simulink model "ParkingMeterSystemNew"  (R2023a)
settings: Solver=FixedStepDiscrete  StartTime=0.0  StopTime=Inf  RelTol=1e-3
PreLoadFcn:
  | % Open the external C# interface
  | startGUI();
PostLoadFcn:
  | warning('off','Simulink:SimulationPacing:UnsupportedSimulationMode');
InitFcn:
  | % Update the sampling time based on the selected simulation mode
  | updateSamplingTime('ParkingMeterSystemNew','SAMPLING_TIME');
undefined symbols (not defined in the file): D1, P
CloseFcn:
  | % Close the external C# interface
  | closeGUI();
settings Model: DataDictionary=Parameters.sldd  Creator=sebas  LastModifiedBy=sebas
settings OptimizationCC: DefaultParameterBehavior=Inlined  EnhancedBackFolding=on  PassReuseOutputArgsAs=Individual arguments  ZeroExternalMemoryAtStartup=off  ZeroInternalMemoryAtStartup=off  OptimizeBlockOrder=speed  DifferentSizesBufferReuse=on  OptimizationCustomize=off  EfficientTunableParamExpr=on
settings DebuggingCC: ParameterTunabilityLossMsg=error
settings SFSimCC: MATLABDynamicMemAlloc=off
settings RTWCC: Description=Embedded Coder  SystemTargetFile=ert.tlc  TemplateMakefile=ert_default_tmf
settings CodeAppCC: ForceParamTrailComments=on  IgnoreCustomStorageClasses=off  MaxIdLength=61  OperatorAnnotations=on  SimulinkDataObjDesc=on  SFDataObjDesc=on  InsertBlockDesc=on
settings ERTTargetCC: TargetLangStandard=C99 (ISO)  GenerateSampleERTMain=on  InlinedParameterPlacement=NonHierarchical  ERTCustomFileTemplate=example_file_process.tlc

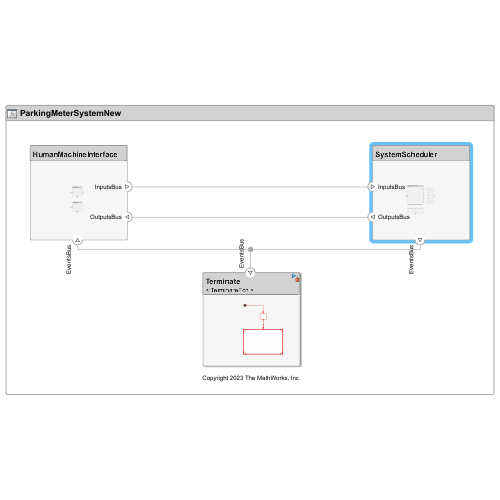
[thumbnail: Simulink's stored preview of the top-level diagram]
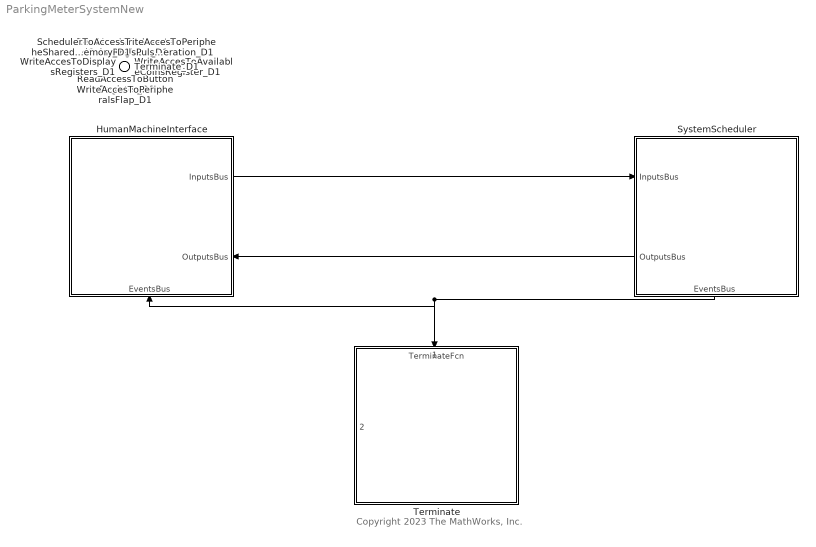
== system ParkingMeterSystemNew ==
  note: Copyright 2023 The MathWorks, Inc.
  ReadAccessToButtonsRegister_D1 : Inport  OutputFunctionCall=on
  ReadAccessToInsertedCoinsRegister_D1 : Inport  Port=2  OutputFunctionCall=on
  WriteAccesToAvailableCoinsRegister_D1 : Inport  Port=3  OutputFunctionCall=on
  WriteAccesToDisplaysRegisters_D1 : Inport  Port=4  OutputFunctionCall=on
  WriteAccesToPeripheralsFlap_D1 : Inport  Port=5  OutputFunctionCall=on
  WriteAccesToPeripheralsPulseGeneration_D1 : Inport  Port=6  OutputFunctionCall=on
  SchedulerToAccessTheSharedMemory_D1 : Inport  Port=7  OutputFunctionCall=on
  Terminate_D1 : Inport  Port=8  OutputFunctionCall=on
  HumanMachineInterface : Subsystem
      settings: PortSchema="{\"entries\":[{\"content\":{\"headerSize\":26,\"margin\":15,\"minimumSpacing\":25,\"sides\":[{\"content\":{},\"type\":\"ConnectorPlacement.EquallySpacedRectSide\",\"uuid\":\"be809503-f1ea-4380-8942-33d79f2ad371\"},{\"content\":{\"connectorIds\":[\"Out1\",\"In2\"],\"side\":\"RIGHT\"},\"type\":\"ConnectorPlacement.EquallySpacedRectSide\",\"uuid\":\"d20c5475-d043-4994-ac49-3eb74728e760\"},{\"content\":{\"side\":\"TOP\"},\"type\":\"ConnectorPlacement.EquallySpacedRectSide\",\"uuid\":\"367a4a40-2fef-41b1-a218-3cfa4d79ed8f\"},{\"content\":{\"connectorIds\":[\"In1\"],\"side\":\"BOTTOM\"},\"type\":\"ConnectorPlacement.EquallySpacedRectSide\",\"uuid\":\"ad45a532-4028-4d32-9ed1-5493ed102a58\"}]},\"type\":\"ConnectorPlacement.EquallySpacedConnector\",\"uuid\":\"eb419f36-354b-4c4e-9a9c-8f8f96d7f82d\"}],\"packageUris\":[\"http://schema.mathworks.com/mf0/Connector/R2020b\"],\"version\":\"1.0\"}"
  SystemScheduler : Subsystem
      settings: PortSchema="{\"entries\":[{\"content\":{\"headerSize\":26,\"margin\":15,\"minimumSpacing\":25,\"sides\":[{\"content\":{\"connectorIds\":[\"In1\",\"Out2\"]},\"type\":\"ConnectorPlacement.EquallySpacedRectSide\",\"uuid\":\"be809503-f1ea-4380-8942-33d79f2ad371\"},{\"content\":{\"side\":\"RIGHT\"},\"type\":\"ConnectorPlacement.EquallySpacedRectSide\",\"uuid\":\"d20c5475-d043-4994-ac49-3eb74728e760\"},{\"content\":{\"side\":\"TOP\"},\"type\":\"ConnectorPlacement.EquallySpacedRectSide\",\"uuid\":\"367a4a40-2fef-41b1-a218-3cfa4d79ed8f\"},{\"content\":{\"connectorIds\":[\"Out1\"],\"side\":\"BOTTOM\"},\"type\":\"ConnectorPlacement.EquallySpacedRectSide\",\"uuid\":\"599a3aa0-021a-4e17-bee6-5fef34730978\"}]},\"type\":\"ConnectorPlacement.EquallySpacedConnector\",\"uuid\":\"eb419f36-354b-4c4e-9a9c-8f8f96d7f82d\"}],\"packageUris\":[\"http://schema.mathworks.com/mf0/Connector/R2020b\"],\"version\":\"1.0\"}"
  Terminate : ModelReference  ModelNameDialog=TerminateFcn  SimulationMode=Normal  ScheduleRates=on  CachedPortDiscreteRates=[0.001]  ModelEventPortInfo=P:D1[0.001][0][0]  ModelReferenceVersion=8.4
      settings: PortSchema="{\"entries\":[{\"content\":{\"headerSize\":38,\"margin\":15,\"minimumSpacing\":25,\"sides\":[{\"content\":{},\"type\":\"ConnectorPlacement.EquallySpacedRectSide\",\"uuid\":\"be809503-f1ea-4380-8942-33d79f2ad371\"},{\"content\":{\"side\":\"RIGHT\"},\"type\":\"ConnectorPlacement.EquallySpacedRectSide\",\"uuid\":\"d20c5475-d043-4994-ac49-3eb74728e760\"},{\"content\":{\"connectorIds\":[\"In1\"],\"side\":\"TOP\"},\"type\":\"ConnectorPlacement.EquallySpacedRectSide\",\"uuid\":\"367a4a40-2fef-41b1-a218-3cfa4d79ed8f\"},{\"content\":{\"connectorIds\":[\"In2\"],\"side\":\"HIDDEN\"},\"type\":\"ConnectorPlacement.EquallySpacedRectSide\",\"uuid\":\"2b7aa608-e8c7-4427-8225-0280e4f358e9\"}]},\"type\":\"ConnectorPlacement.EquallySpacedConnector\",\"uuid\":\"eb419f36-354b-4c4e-9a9c-8f8f96d7f82d\"}],\"packageUris\":[\"http://schema.mathworks.com/mf0/Connector/R2020b\"],\"version\":\"1.0\"}"
  wires:
  SystemScheduler/2(OutputsBus) -> HumanMachineInterface/2(OutputsBus)
  HumanMachineInterface/1(InputsBus) -> SystemScheduler/1(InputsBus)
  SystemScheduler/1(EventsBus) -> Terminate/1, HumanMachineInterface/1(EventsBus)

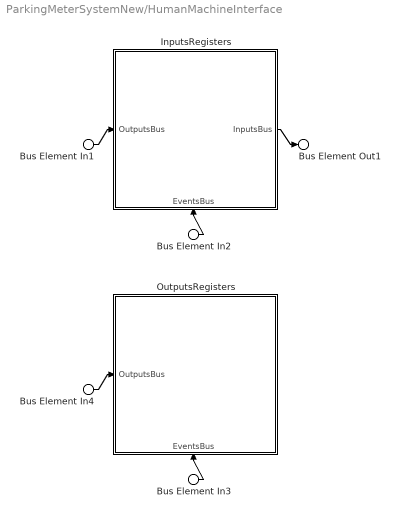
== system ParkingMeterSystemNew/HumanMachineInterface ==
  Bus Element In2 : Inport  PortName=EventsBus
  Bus Element In3 : Inport  PortName=EventsBus
  Bus Element In1 : Inport  Port=2  PortName=OutputsBus
  Bus Element In4 : Inport  Port=2  PortName=OutputsBus
  InputsRegisters : Subsystem
      settings: PortSchema="{\"entries\":[{\"content\":{\"headerSize\":26,\"margin\":15,\"minimumSpacing\":25,\"sides\":[{\"content\":{\"connectorIds\":[\"In2\"]},\"type\":\"ConnectorPlacement.EquallySpacedRectSide\",\"uuid\":\"be809503-f1ea-4380-8942-33d79f2ad371\"},{\"content\":{\"connectorIds\":[\"Out1\"],\"side\":\"RIGHT\"},\"type\":\"ConnectorPlacement.EquallySpacedRectSide\",\"uuid\":\"d20c5475-d043-4994-ac49-3eb74728e760\"},{\"content\":{\"side\":\"TOP\"},\"type\":\"ConnectorPlacement.EquallySpacedRectSide\",\"uuid\":\"367a4a40-2fef-41b1-a218-3cfa4d79ed8f\"},{\"content\":{\"connectorIds\":[\"In1\"],\"side\":\"BOTTOM\"},\"type\":\"ConnectorPlacement.EquallySpacedRectSide\",\"uuid\":\"42433694-7d38-411e-8c36-0d107f91df78\"}]},\"type\":\"ConnectorPlacement.EquallySpacedConnector\",\"uuid\":\"eb419f36-354b-4c4e-9a9c-8f8f96d7f82d\"}],\"packageUris\":[\"http://schema.mathworks.com/mf0/Connector/R2020b\"],\"version\":\"1.0\"}"
  OutputsRegisters : Subsystem
      settings: PortSchema="{\"entries\":[{\"content\":{\"headerSize\":26,\"margin\":15,\"minimumSpacing\":25,\"sides\":[{\"content\":{\"connectorIds\":[\"In1\"]},\"type\":\"ConnectorPlacement.EquallySpacedRectSide\",\"uuid\":\"be809503-f1ea-4380-8942-33d79f2ad371\"},{\"content\":{\"side\":\"RIGHT\"},\"type\":\"ConnectorPlacement.EquallySpacedRectSide\",\"uuid\":\"d20c5475-d043-4994-ac49-3eb74728e760\"},{\"content\":{\"side\":\"TOP\"},\"type\":\"ConnectorPlacement.EquallySpacedRectSide\",\"uuid\":\"367a4a40-2fef-41b1-a218-3cfa4d79ed8f\"},{\"content\":{\"connectorIds\":[\"In2\"],\"side\":\"BOTTOM\"},\"type\":\"ConnectorPlacement.EquallySpacedRectSide\",\"uuid\":\"9411f4e0-b09e-492c-9d7b-7970a952076c\"}]},\"type\":\"ConnectorPlacement.EquallySpacedConnector\",\"uuid\":\"eb419f36-354b-4c4e-9a9c-8f8f96d7f82d\"}],\"packageUris\":[\"http://schema.mathworks.com/mf0/Connector/R2020b\"],\"version\":\"1.0\"}"
  Bus Element Out1 : Outport  PortName=InputsBus
  wires:
  Bus Element In1/1 -> InputsRegisters/2(OutputsBus)
  InputsRegisters/1(InputsBus) -> Bus Element Out1/1
  Bus Element In2/1 -> InputsRegisters/1(EventsBus)
  Bus Element In3/1 -> OutputsRegisters/2(EventsBus)
  Bus Element In4/1 -> OutputsRegisters/1(OutputsBus)

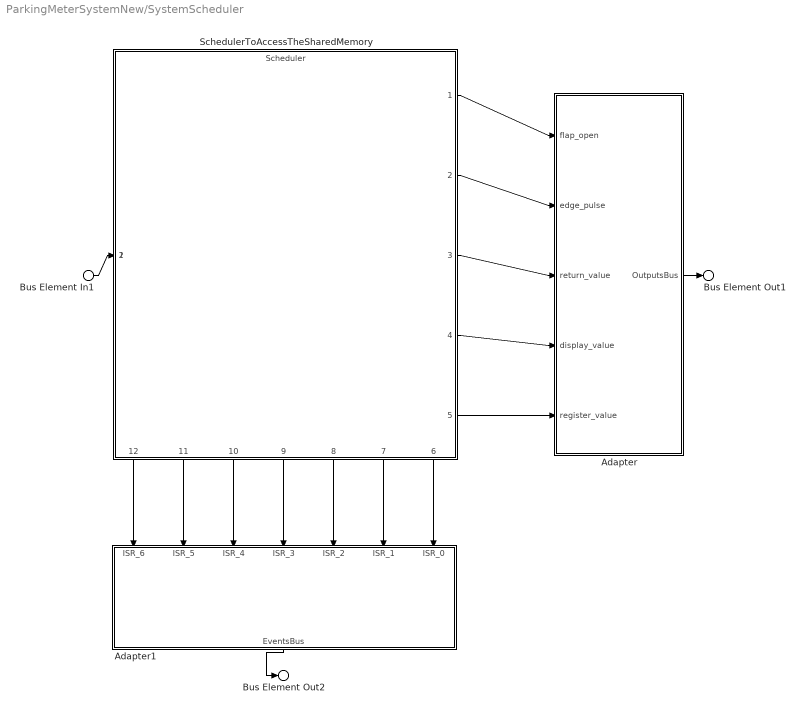
== system ParkingMeterSystemNew/SystemScheduler ==
  Bus Element In1 : Inport  PortName=InputsBus
  Adapter : Subsystem
      settings: PortSchema="{\"entries\":[{\"content\":{\"margin\":10,\"minimumSpacing\":15,\"sides\":[{\"content\":{\"connectorIds\":[\"In1\",\"In2\",\"In3\",\"In4\",\"In5\"]},\"type\":\"ConnectorPlacement.EquallySpacedRectSide\",\"uuid\":\"be809503-f1ea-4380-8942-33d79f2ad371\"},{\"content\":{\"connectorIds\":[\"Out1\"],\"side\":\"RIGHT\"},\"type\":\"ConnectorPlacement.EquallySpacedRectSide\",\"uuid\":\"d20c5475-d043-4994-ac49-3eb74728e760\"},{\"content\":{\"side\":\"TOP\"},\"type\":\"ConnectorPlacement.EquallySpacedRectSide\",\"uuid\":\"367a4a40-2fef-41b1-a218-3cfa4d79ed8f\"}]},\"type\":\"ConnectorPlacement.EquallySpacedConnector\",\"uuid\":\"eb419f36-354b-4c4e-9a9c-8f8f96d7f82d\"}],\"packageUris\":[\"http://schema.mathworks.com/mf0/Connector/R2020b\"],\"version\":\"1.0\"}"
  Adapter1 : Subsystem
      settings: PortSchema="{\"entries\":[{\"content\":{\"margin\":10,\"minimumSpacing\":15,\"sides\":[{\"content\":{},\"type\":\"ConnectorPlacement.EquallySpacedRectSide\",\"uuid\":\"be809503-f1ea-4380-8942-33d79f2ad371\"},{\"content\":{\"side\":\"RIGHT\"},\"type\":\"ConnectorPlacement.EquallySpacedRectSide\",\"uuid\":\"d20c5475-d043-4994-ac49-3eb74728e760\"},{\"content\":{\"connectorIds\":[\"In1\",\"In2\",\"In3\",\"In4\",\"In5\",\"In6\",\"In7\"],\"side\":\"TOP\"},\"type\":\"ConnectorPlacement.EquallySpacedRectSide\",\"uuid\":\"367a4a40-2fef-41b1-a218-3cfa4d79ed8f\"},{\"content\":{\"connectorIds\":[\"Out1\"],\"side\":\"BOTTOM\"},\"type\":\"ConnectorPlacement.EquallySpacedRectSide\",\"uuid\":\"de1afc0c-f7fe-45f0-a616-bbe694a265ab\"}]},\"type\":\"ConnectorPlacement.EquallySpacedConnector\",\"uuid\":\"eb419f36-354b-4c4e-9a9c-8f8f96d7f82d\"}],\"packageUris\":[\"http://schema.mathworks.com/mf0/Connector/R2020b\"],\"version\":\"1.0\"}"
  SchedulerToAccessTheSharedMemory : ModelReference  ModelNameDialog=Scheduler  SimulationMode=Normal  ScheduleRates=on  CachedPortDiscreteRates=[0.001]  ModelEventPortInfo=P:D1[0.001][0][0]  ModelReferenceVersion=8.3
      settings: PortSchema="{\"entries\":[{\"content\":{\"headerSize\":38,\"margin\":15,\"minimumSpacing\":25,\"sides\":[{\"content\":{\"connectorIds\":[\"In1\"]},\"type\":\"ConnectorPlacement.EquallySpacedRectSide\",\"uuid\":\"be809503-f1ea-4380-8942-33d79f2ad371\"},{\"content\":{\"connectorIds\":[\"Out1\",\"Out2\",\"Out3\",\"Out4\",\"Out5\"],\"side\":\"RIGHT\"},\"type\":\"ConnectorPlacement.EquallySpacedRectSide\",\"uuid\":\"d20c5475-d043-4994-ac49-3eb74728e760\"},{\"content\":{\"side\":\"TOP\"},\"type\":\"ConnectorPlacement.EquallySpacedRectSide\",\"uuid\":\"367a4a40-2fef-41b1-a218-3cfa4d79ed8f\"},{\"content\":{\"connectorIds\":[\"Out12\",\"Out11\",\"Out10\",\"Out9\",\"Out8\",\"Out7\",\"Out6\"],\"side\":\"BOTTOM\"},\"type\":\"ConnectorPlacement.EquallySpacedRectSide\",\"uuid\":\"fb86e00b-f9c7-4f3f-8cbd-dd4de8ac92df\"},{\"content\":{\"connectorIds\":[\"In2\"],\"side\":\"HIDDEN\"},\"type\":\"ConnectorPlacement.EquallySpacedRectSide\",\"uuid\":\"74e265bb-5a4f-4039-8bd9-f78af680f503\"}]},\"type\":\"ConnectorPlacement.EquallySpacedConnector\",\"uuid\":\"eb419f36-354b-4c4e-9a9c-8f8f96d7f82d\"}],\"packageUris\":[\"http://schema.mathworks.com/mf0/Connector/R2020b\"],\"version\":\"1.0\"}"
  Bus Element Out2 : Outport  PortName=EventsBus
  Bus Element Out1 : Outport  Port=2  PortName=OutputsBus
  wires:
  Adapter/1(OutputsBus) -> Bus Element Out1/1
  SchedulerToAccessTheSharedMemory/1 -> Adapter/1(flap_open)
  SchedulerToAccessTheSharedMemory/2 -> Adapter/2(edge_pulse)
  SchedulerToAccessTheSharedMemory/3 -> Adapter/3(return_value)
  SchedulerToAccessTheSharedMemory/4 -> Adapter/4(display_value)
  SchedulerToAccessTheSharedMemory/5 -> Adapter/5(register_value)
  Adapter1/1(EventsBus) -> Bus Element Out2/1
  SchedulerToAccessTheSharedMemory/12 -> Adapter1/1(ISR_6)
  SchedulerToAccessTheSharedMemory/11 -> Adapter1/2(ISR_5)
  SchedulerToAccessTheSharedMemory/10 -> Adapter1/3(ISR_4)
  SchedulerToAccessTheSharedMemory/9 -> Adapter1/4(ISR_3)
  SchedulerToAccessTheSharedMemory/8 -> Adapter1/5(ISR_2)
  SchedulerToAccessTheSharedMemory/7 -> Adapter1/6(ISR_1)
  SchedulerToAccessTheSharedMemory/6 -> Adapter1/7(ISR_0)
  Bus Element In1/1 -> SchedulerToAccessTheSharedMemory/1

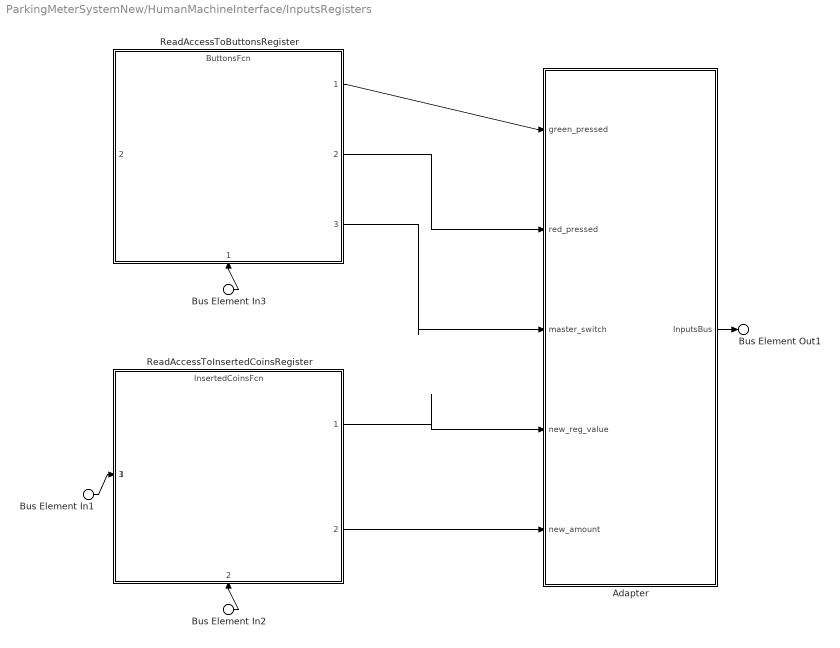
== system ParkingMeterSystemNew/HumanMachineInterface/InputsRegisters ==
  Bus Element In2 : Inport  PortName=EventsBus
  Bus Element In3 : Inport  PortName=EventsBus
  Bus Element In1 : Inport  Port=2  PortName=OutputsBus
  Adapter : Subsystem
      settings: PortSchema="{\"entries\":[{\"content\":{\"margin\":10,\"minimumSpacing\":15,\"sides\":[{\"content\":{\"connectorIds\":[\"In1\",\"In2\",\"In3\",\"In4\",\"In5\"]},\"type\":\"ConnectorPlacement.EquallySpacedRectSide\",\"uuid\":\"be809503-f1ea-4380-8942-33d79f2ad371\"},{\"content\":{\"connectorIds\":[\"Out1\"],\"side\":\"RIGHT\"},\"type\":\"ConnectorPlacement.EquallySpacedRectSide\",\"uuid\":\"d20c5475-d043-4994-ac49-3eb74728e760\"},{\"content\":{\"side\":\"TOP\"},\"type\":\"ConnectorPlacement.EquallySpacedRectSide\",\"uuid\":\"367a4a40-2fef-41b1-a218-3cfa4d79ed8f\"}]},\"type\":\"ConnectorPlacement.EquallySpacedConnector\",\"uuid\":\"eb419f36-354b-4c4e-9a9c-8f8f96d7f82d\"}],\"packageUris\":[\"http://schema.mathworks.com/mf0/Connector/R2020b\"],\"version\":\"1.0\"}"
  ReadAccessToButtonsRegister : ModelReference  ModelNameDialog=ButtonsFcn  SimulationMode=Normal  ScheduleRates=on  CachedPortDiscreteRates=[0.001]  ModelEventPortInfo=P:D1[0.001][0][0]  ModelReferenceVersion=8.1
      settings: PortSchema="{\"entries\":[{\"content\":{\"headerSize\":38,\"margin\":15,\"minimumSpacing\":25,\"sides\":[{\"content\":{},\"type\":\"ConnectorPlacement.EquallySpacedRectSide\",\"uuid\":\"be809503-f1ea-4380-8942-33d79f2ad371\"},{\"content\":{\"connectorIds\":[\"Out1\",\"Out2\",\"Out3\"],\"side\":\"RIGHT\"},\"type\":\"ConnectorPlacement.EquallySpacedRectSide\",\"uuid\":\"d20c5475-d043-4994-ac49-3eb74728e760\"},{\"content\":{\"side\":\"TOP\"},\"type\":\"ConnectorPlacement.EquallySpacedRectSide\",\"uuid\":\"367a4a40-2fef-41b1-a218-3cfa4d79ed8f\"},{\"content\":{\"connectorIds\":[\"In1\"],\"side\":\"BOTTOM\"},\"type\":\"ConnectorPlacement.EquallySpacedRectSide\",\"uuid\":\"20a3fabb-dc20-4c8a-b758-ffeffe12cb5d\"},{\"content\":{\"connectorIds\":[\"In2\"],\"side\":\"HIDDEN\"},\"type\":\"ConnectorPlacement.EquallySpacedRectSide\",\"uuid\":\"619db0d7-0664-4085-915a-a74ff553ccfa\"}]},\"type\":\"ConnectorPlacement.EquallySpacedConnector\",\"uuid\":\"eb419f36-354b-4c4e-9a9c-8f8f96d7f82d\"}],\"packageUris\":[\"http://schema.mathworks.com/mf0/Connector/R2020b\"],\"version\":\"1.0\"}"
  ReadAccessToInsertedCoinsRegister : ModelReference  ModelNameDialog=InsertedCoinsFcn  SimulationMode=Normal  ScheduleRates=on  CachedPortDiscreteRates=[0.001]  ModelEventPortInfo=P:D1[0.001][0][0]  ModelReferenceVersion=8.4
      settings: PortSchema="{\"entries\":[{\"content\":{\"headerSize\":38,\"margin\":15,\"minimumSpacing\":25,\"sides\":[{\"content\":{\"connectorIds\":[\"In1\"]},\"type\":\"ConnectorPlacement.EquallySpacedRectSide\",\"uuid\":\"be809503-f1ea-4380-8942-33d79f2ad371\"},{\"content\":{\"connectorIds\":[\"Out1\",\"Out2\"],\"side\":\"RIGHT\"},\"type\":\"ConnectorPlacement.EquallySpacedRectSide\",\"uuid\":\"d20c5475-d043-4994-ac49-3eb74728e760\"},{\"content\":{\"side\":\"TOP\"},\"type\":\"ConnectorPlacement.EquallySpacedRectSide\",\"uuid\":\"367a4a40-2fef-41b1-a218-3cfa4d79ed8f\"},{\"content\":{\"connectorIds\":[\"In2\"],\"side\":\"BOTTOM\"},\"type\":\"ConnectorPlacement.EquallySpacedRectSide\",\"uuid\":\"c4a18945-d859-4bf0-a176-342256d1a336\"},{\"content\":{\"connectorIds\":[\"In3\"],\"side\":\"HIDDEN\"},\"type\":\"ConnectorPlacement.EquallySpacedRectSide\",\"uuid\":\"52804af8-db2a-4760-b62b-c289e870e5aa\"}]},\"type\":\"ConnectorPlacement.EquallySpacedConnector\",\"uuid\":\"eb419f36-354b-4c4e-9a9c-8f8f96d7f82d\"}],\"packageUris\":[\"http://schema.mathworks.com/mf0/Connector/R2020b\"],\"version\":\"1.0\"}"
  Bus Element Out1 : Outport  PortName=InputsBus
  wires:
  Bus Element In1/1 -> ReadAccessToInsertedCoinsRegister/1
  Bus Element In2/1 -> ReadAccessToInsertedCoinsRegister/2
  Bus Element In3/1 -> ReadAccessToButtonsRegister/1
  Adapter/1(InputsBus) -> Bus Element Out1/1
  ReadAccessToButtonsRegister/1 -> Adapter/1(green_pressed)
  ReadAccessToButtonsRegister/2 -> Adapter/2(red_pressed)
  ReadAccessToButtonsRegister/3 -> Adapter/3(master_switch)
  ReadAccessToInsertedCoinsRegister/1 -> Adapter/4(new_reg_value)
  ReadAccessToInsertedCoinsRegister/2 -> Adapter/5(new_amount)

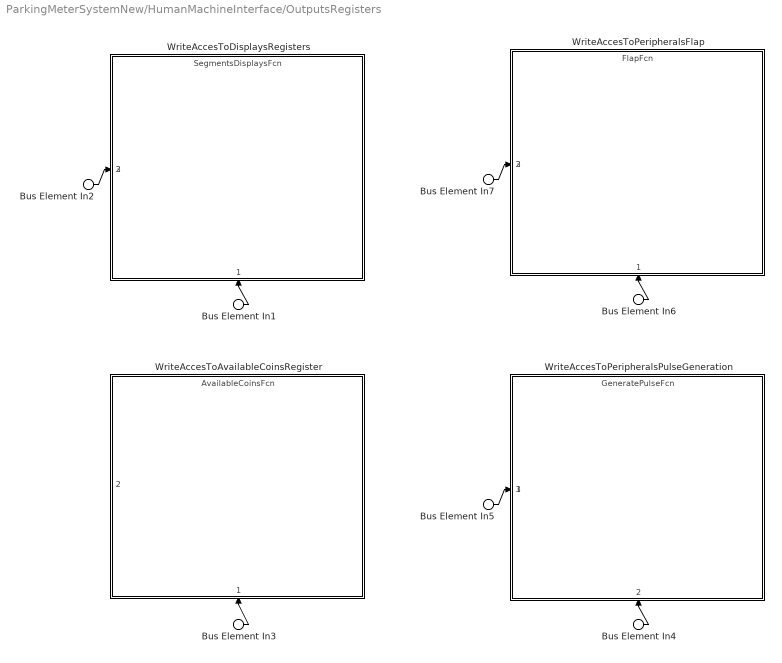
== system ParkingMeterSystemNew/HumanMachineInterface/OutputsRegisters ==
  Bus Element In2 : Inport  PortName=OutputsBus
  Bus Element In5 : Inport  PortName=OutputsBus
  Bus Element In7 : Inport  PortName=OutputsBus
  Bus Element In{1,3..4,6} (4 alike) : Inport  Port=2  PortName=EventsBus
  WriteAccesToAvailableCoinsRegister : ModelReference  ModelNameDialog=AvailableCoinsFcn  SimulationMode=Normal  ScheduleRates=on  CachedPortDiscreteRates=[0.001]  ModelEventPortInfo=P:D1[0.001][0][0]  ModelReferenceVersion=8.4
      settings: PortSchema="{\"entries\":[{\"content\":{\"headerSize\":38,\"margin\":15,\"minimumSpacing\":25,\"sides\":[{\"content\":{},\"type\":\"ConnectorPlacement.EquallySpacedRectSide\",\"uuid\":\"be809503-f1ea-4380-8942-33d79f2ad371\"},{\"content\":{\"side\":\"RIGHT\"},\"type\":\"ConnectorPlacement.EquallySpacedRectSide\",\"uuid\":\"d20c5475-d043-4994-ac49-3eb74728e760\"},{\"content\":{\"side\":\"TOP\"},\"type\":\"ConnectorPlacement.EquallySpacedRectSide\",\"uuid\":\"367a4a40-2fef-41b1-a218-3cfa4d79ed8f\"},{\"content\":{\"connectorIds\":[\"In1\"],\"side\":\"BOTTOM\"},\"type\":\"ConnectorPlacement.EquallySpacedRectSide\",\"uuid\":\"0ec21bd5-d732-4e1f-9584-045b5c892f8a\"},{\"content\":{\"connectorIds\":[\"In2\"],\"side\":\"HIDDEN\"},\"type\":\"ConnectorPlacement.EquallySpacedRectSide\",\"uuid\":\"3eb33428-824a-4da5-832a-2eacaca34f61\"}]},\"type\":\"ConnectorPlacement.EquallySpacedConnector\",\"uuid\":\"eb419f36-354b-4c4e-9a9c-8f8f96d7f82d\"}],\"packageUris\":[\"http://schema.mathworks.com/mf0/Connector/R2020b\"],\"version\":\"1.0\"}"
  WriteAccesToDisplaysRegisters : ModelReference  ModelNameDialog=SegmentsDisplaysFcn  SimulationMode=Normal  ScheduleRates=on  CachedPortDiscreteRates=[0.001]  ModelEventPortInfo=P:D1[0.001][0][0]  ModelReferenceVersion=8.4
      settings: PortSchema="{\"entries\":[{\"content\":{\"headerSize\":38,\"margin\":15,\"minimumSpacing\":25,\"sides\":[{\"content\":{\"connectorIds\":[\"In2\"]},\"type\":\"ConnectorPlacement.EquallySpacedRectSide\",\"uuid\":\"be809503-f1ea-4380-8942-33d79f2ad371\"},{\"content\":{\"side\":\"RIGHT\"},\"type\":\"ConnectorPlacement.EquallySpacedRectSide\",\"uuid\":\"d20c5475-d043-4994-ac49-3eb74728e760\"},{\"content\":{\"side\":\"TOP\"},\"type\":\"ConnectorPlacement.EquallySpacedRectSide\",\"uuid\":\"367a4a40-2fef-41b1-a218-3cfa4d79ed8f\"},{\"content\":{\"connectorIds\":[\"In1\"],\"side\":\"BOTTOM\"},\"type\":\"ConnectorPlacement.EquallySpacedRectSide\",\"uuid\":\"41896e6e-9ee0-46f4-85c5-427c3971bd92\"},{\"content\":{\"connectorIds\":[\"In3\"],\"side\":\"HIDDEN\"},\"type\":\"ConnectorPlacement.EquallySpacedRectSide\",\"uuid\":\"0339ac93-600c-466f-8072-11d736857049\"}]},\"type\":\"ConnectorPlacement.EquallySpacedConnector\",\"uuid\":\"eb419f36-354b-4c4e-9a9c-8f8f96d7f82d\"}],\"packageUris\":[\"http://schema.mathworks.com/mf0/Connector/R2020b\"],\"version\":\"1.0\"}"
  WriteAccesToPeripheralsFlap : ModelReference  ModelNameDialog=FlapFcn  SimulationMode=Normal  ScheduleRates=on  CachedPortDiscreteRates=[0.001]  ModelEventPortInfo=P:D1[0.001][0][0]  ModelReferenceVersion=8.4
      settings: PortSchema="{\"entries\":[{\"content\":{\"headerSize\":38,\"margin\":15,\"minimumSpacing\":25,\"sides\":[{\"content\":{\"connectorIds\":[\"In2\"]},\"type\":\"ConnectorPlacement.EquallySpacedRectSide\",\"uuid\":\"be809503-f1ea-4380-8942-33d79f2ad371\"},{\"content\":{\"side\":\"RIGHT\"},\"type\":\"ConnectorPlacement.EquallySpacedRectSide\",\"uuid\":\"d20c5475-d043-4994-ac49-3eb74728e760\"},{\"content\":{\"side\":\"TOP\"},\"type\":\"ConnectorPlacement.EquallySpacedRectSide\",\"uuid\":\"367a4a40-2fef-41b1-a218-3cfa4d79ed8f\"},{\"content\":{\"connectorIds\":[\"In1\"],\"side\":\"BOTTOM\"},\"type\":\"ConnectorPlacement.EquallySpacedRectSide\",\"uuid\":\"14e3096b-a6b9-4981-8345-e34eabc07420\"},{\"content\":{\"connectorIds\":[\"In3\"],\"side\":\"HIDDEN\"},\"type\":\"ConnectorPlacement.EquallySpacedRectSide\",\"uuid\":\"98d0f007-bbbb-419c-9a0b-eb95b9f54b7b\"}]},\"type\":\"ConnectorPlacement.EquallySpacedConnector\",\"uuid\":\"eb419f36-354b-4c4e-9a9c-8f8f96d7f82d\"}],\"packageUris\":[\"http://schema.mathworks.com/mf0/Connector/R2020b\"],\"version\":\"1.0\"}"
  WriteAccesToPeripheralsPulseGeneration : ModelReference  ModelNameDialog=GeneratePulseFcn  SimulationMode=Normal  ScheduleRates=on  CachedPortDiscreteRates=[0.15]  ModelEventPortInfo=P:D1[0.15][0][0]  ModelReferenceVersion=8.4
      settings: PortSchema="{\"entries\":[{\"content\":{\"headerSize\":38,\"margin\":15,\"minimumSpacing\":25,\"sides\":[{\"content\":{\"connectorIds\":[\"In1\"]},\"type\":\"ConnectorPlacement.EquallySpacedRectSide\",\"uuid\":\"be809503-f1ea-4380-8942-33d79f2ad371\"},{\"content\":{\"side\":\"RIGHT\"},\"type\":\"ConnectorPlacement.EquallySpacedRectSide\",\"uuid\":\"d20c5475-d043-4994-ac49-3eb74728e760\"},{\"content\":{\"side\":\"TOP\"},\"type\":\"ConnectorPlacement.EquallySpacedRectSide\",\"uuid\":\"367a4a40-2fef-41b1-a218-3cfa4d79ed8f\"},{\"content\":{\"connectorIds\":[\"In2\"],\"side\":\"BOTTOM\"},\"type\":\"ConnectorPlacement.EquallySpacedRectSide\",\"uuid\":\"a191c519-7795-4009-b1e2-432976e0f9f0\"},{\"content\":{\"connectorIds\":[\"In3\"],\"side\":\"HIDDEN\"},\"type\":\"ConnectorPlacement.EquallySpacedRectSide\",\"uuid\":\"c29be4a7-1c06-4825-ad5a-289e3e32d959\"}]},\"type\":\"ConnectorPlacement.EquallySpacedConnector\",\"uuid\":\"eb419f36-354b-4c4e-9a9c-8f8f96d7f82d\"}],\"packageUris\":[\"http://schema.mathworks.com/mf0/Connector/R2020b\"],\"version\":\"1.0\"}"
  wires:
  Bus Element In2/1 -> WriteAccesToDisplaysRegisters/2
  Bus Element In1/1 -> WriteAccesToDisplaysRegisters/1
  Bus Element In3/1 -> WriteAccesToAvailableCoinsRegister/1
  Bus Element In4/1 -> WriteAccesToPeripheralsPulseGeneration/2
  Bus Element In5/1 -> WriteAccesToPeripheralsPulseGeneration/1
  Bus Element In6/1 -> WriteAccesToPeripheralsFlap/1
  Bus Element In7/1 -> WriteAccesToPeripheralsFlap/2

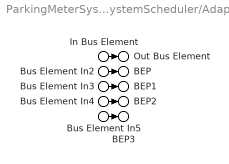
== system ParkingMeterSystemNew/SystemScheduler/Adapter ==
  In Bus Element : Inport  PortName=flap_open
  Bus Element In2 : Inport  Port=2  PortName=edge_pulse
  Bus Element In3 : Inport  Port=3  PortName=return_value
  Bus Element In4 : Inport  Port=4  PortName=display_value
  Bus Element In5 : Inport  Port=5  PortName=register_value
  Out Bus Element : Outport  PortName=OutputsBus  Element=flap_open
  BEP : Outport  PortName=OutputsBus  Element=edge_pulse
  BEP1 : Outport  PortName=OutputsBus  Element=return_value
  BEP2 : Outport  PortName=OutputsBus  Element=display_value
  BEP3 : Outport  PortName=OutputsBus  Element=register_value
  wires:
  In Bus Element/1 -> Out Bus Element/1
  Bus Element In2/1 -> BEP/1
  Bus Element In3/1 -> BEP1/1
  Bus Element In4/1 -> BEP2/1
  Bus Element In5/1 -> BEP3/1

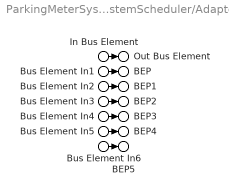
== system ParkingMeterSystemNew/SystemScheduler/Adapter1 ==
  Bus Element In6 : Inport  PortName=ISR_6
  Bus Element In5 : Inport  Port=2  PortName=ISR_5
  Bus Element In4 : Inport  Port=3  PortName=ISR_4
  Bus Element In3 : Inport  Port=4  PortName=ISR_3
  Bus Element In2 : Inport  Port=5  PortName=ISR_2
  Bus Element In1 : Inport  Port=6  PortName=ISR_1
  In Bus Element : Inport  Port=7  PortName=ISR_0
  Out Bus Element : Outport  PortName=EventsBus  Element=ISR_0
  BEP : Outport  PortName=EventsBus  Element=ISR_1
  BEP1 : Outport  PortName=EventsBus  Element=ISR_2
  BEP2 : Outport  PortName=EventsBus  Element=ISR_3
  BEP3 : Outport  PortName=EventsBus  Element=ISR_4
  BEP4 : Outport  PortName=EventsBus  Element=ISR_5
  BEP5 : Outport  PortName=EventsBus  Element=ISR_6
  wires:
  In Bus Element/1 -> Out Bus Element/1
  Bus Element In1/1 -> BEP/1
  Bus Element In2/1 -> BEP1/1
  Bus Element In3/1 -> BEP2/1
  Bus Element In4/1 -> BEP3/1
  Bus Element In5/1 -> BEP4/1
  Bus Element In6/1 -> BEP5/1

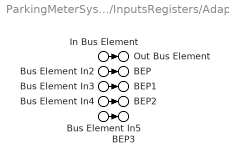
== system ParkingMeterSystemNew/HumanMachineInterface/InputsRegisters/Adapter ==
  In Bus Element : Inport  PortName=green_pressed
  Bus Element In2 : Inport  Port=2  PortName=red_pressed
  Bus Element In3 : Inport  Port=3  PortName=master_switch
  Bus Element In4 : Inport  Port=4  PortName=new_reg_value
  Bus Element In5 : Inport  Port=5  PortName=new_amount
  Out Bus Element : Outport  PortName=InputsBus  Element=green_pressed
  BEP : Outport  PortName=InputsBus  Element=red_pressed
  BEP1 : Outport  PortName=InputsBus  Element=master_switch
  BEP2 : Outport  PortName=InputsBus  Element=coins_reg_value
  BEP3 : Outport  PortName=InputsBus  Element=temp_amount
  wires:
  In Bus Element/1 -> Out Bus Element/1
  Bus Element In2/1 -> BEP/1
  Bus Element In3/1 -> BEP1/1
  Bus Element In4/1 -> BEP2/1
  Bus Element In5/1 -> BEP3/1
